simulink model "testVPSdriver"  (R2015b)
settings: Solver=VariableStepAuto  StartTime=0.0  StopTime=inf  RelTol=1e-3
libraries: robotlib x2
settings Model: Creator=exbot  LastModifiedBy=exbot

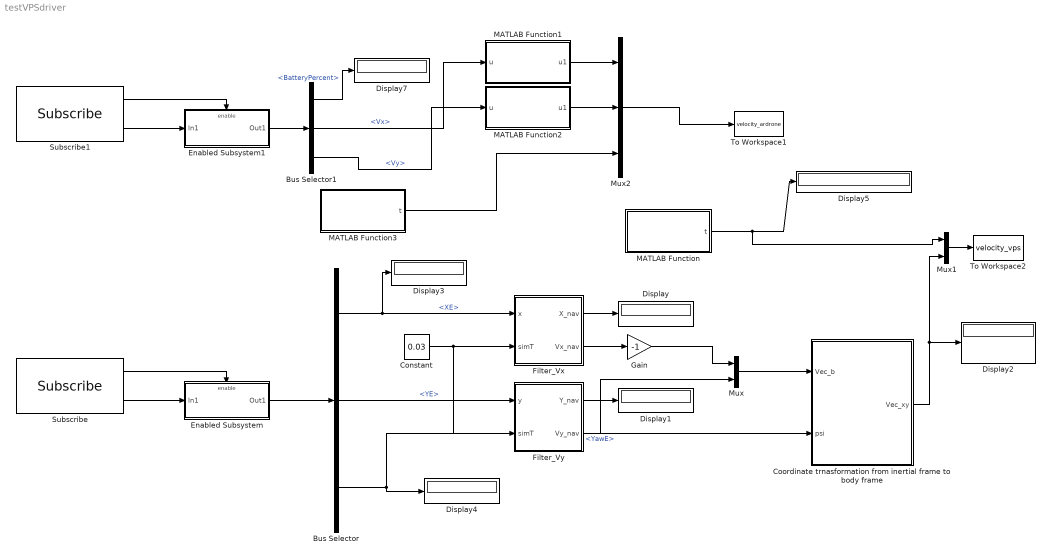
== system testVPSdriver ==
  Bus Selector : BusSelector  OutputSignals=XE,YE,YawE
  Bus Selector1 : BusSelector  OutputSignals=BatteryPercent,Vx,Vy
  Constant : Constant  Value=0.03
  "Coordinate trnasformation from inertial frame to body frame " : MATLAB Function  TreatAsAtomicUnit=on
  Display{,1..5,7} (7 alike) : Display
  Enabled Subsystem : Subsystem  TreatAsAtomicUnit=on
  Enabled Subsystem1 : Subsystem  TreatAsAtomicUnit=on
  Filter_Vx : MATLAB Function  TreatAsAtomicUnit=on
  Filter_Vy : MATLAB Function  TreatAsAtomicUnit=on
  Gain : Gain  Gain=-1
  MATLAB Function : MATLAB Function  TreatAsAtomicUnit=on
  MATLAB Function1 : MATLAB Function  TreatAsAtomicUnit=on
  MATLAB Function2 : MATLAB Function  TreatAsAtomicUnit=on
  MATLAB Function3 : MATLAB Function  TreatAsAtomicUnit=on
  Mux : Mux  Inputs=2
  Mux1 : Mux  Inputs=2
  Mux2 : Mux  Inputs=3
  Subscribe : robotlib/Subscribe  SourceLibraryInfo=This block requires Robotics System Toolbox  topicSource=Select from ROS network  topic=/vpsnavdata  messageType=vps_driver/vps_navdata  sampleTime=-1  messageQueueLength=1
  Subscribe1 : robotlib/Subscribe  SourceLibraryInfo=This block requires Robotics System Toolbox  topicSource=Select from ROS network  topic=/ardrone/navdata  messageType=ardrone_autonomy/Navdata  sampleTime=-1  messageQueueLength=1
  To Workspace1 : ToWorkspace  VariableName=velocity_ardrone  SampleTime=-1
  To Workspace2 : ToWorkspace  VariableName=velocity_vps  SampleTime=-1
  wires:
  Subscribe/2 -> Enabled Subsystem/1(In1)
  Subscribe/1 -> Enabled Subsystem/Enable
  Bus Selector/1 -> Display3/1, Filter_Vx/1(x)  "<XE>"
  Bus Selector/2 -> Filter_Vy/1(y)  "<YE>"
  Enabled Subsystem/1(Out1) -> Bus Selector/1
  Subscribe1/2 -> Enabled Subsystem1/1(In1)
  Subscribe1/1 -> Enabled Subsystem1/Enable
  Enabled Subsystem1/1(Out1) -> Bus Selector1/1
  Bus Selector1/1 -> Display7/1  "<BatteryPercent>"
  Bus Selector1/2 -> MATLAB Function1/1(u)  "<Vx>"
  Bus Selector1/3 -> MATLAB Function2/1(u)  "<Vy>"
  Mux2/1 -> To Workspace1/1
  Bus Selector/3 -> "Coordinate trnasformation from inertial frame to body frame "/2(psi), Display4/1  "<YawE>"
  Filter_Vx/1(X_nav) -> Display/1
  Filter_Vy/1(Y_nav) -> Display1/1
  Mux/1 -> "Coordinate trnasformation from inertial frame to body frame "/1(Vec_b)
  Filter_Vx/2(Vx_nav) -> Gain/1
  Filter_Vy/2(Vy_nav) -> Mux/2
  Constant/1 -> Filter_Vy/2(simT), Filter_Vx/2(simT)
  MATLAB Function/1(t) -> Mux1/1, Display5/1
  "Coordinate trnasformation from inertial frame to body frame "/1(Vec_xy) -> Mux1/2, Display2/1
  Mux1/1 -> To Workspace2/1
  MATLAB Function3/1(t) -> Mux2/3
  MATLAB Function1/1(u1) -> Mux2/1
  MATLAB Function2/1(u1) -> Mux2/2
  Gain/1 -> Mux/1

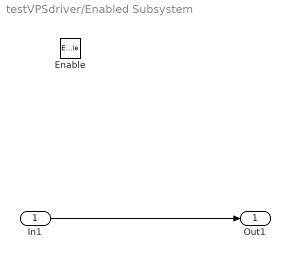
== system testVPSdriver/Enabled Subsystem ==
  In1 : Inport
  Enable : EnablePort
  Out1 : Outport
  wires:
  In1/1 -> Out1/1

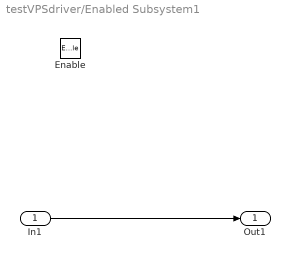
== system testVPSdriver/Enabled Subsystem1 ==
  In1 : Inport
  Enable : EnablePort
  Out1 : Outport
  wires:
  In1/1 -> Out1/1

== matlab function testVPSdriver/Coordinate trnasformation from inertial frame to body frame  ==
  data: Vec_b input; Vec_xy output; psi input
function Vec_xy  = fcn(Vec_b , psi)
%#codegen
T = [cos(psi) sin(psi) ; sin(psi) -cos(psi)] ; 
Vec_xy = T*Vec_b(1:2,1);

== matlab function testVPSdriver/MATLAB Function ==
  data: t output
function t = sysTime( )
coder.extrinsic('now');
t = 0;
t = now;
end

== matlab function testVPSdriver/Filter_Vx ==
  data: x input; X_nav output; Vx_nav output; simT input
function [X_nav,Vx_nav] = fcn(x,simT)
persistent Phi;
if isempty(Phi)
    Phi = [1 simT;0 1];
end

persistent Tao;
if isempty(Tao)
    Tao = [0 simT]';
end

persistent Q;
if isempty(Q)
    Q = 50;
end

persistent H;
if isempty(H)
    H = [1 0];
end

persistent R;
if isempty(R)
    R = 7.81e-1;
end

persistent Xe;
if isempty(Xe)
    Xe = [0 0]';
end

persistent X_e;
if isempty(X_e)
    X_e = [0 0]';
end

persistent Z_e;
if isempty(Z_e)
    Z_e = 0;
end

persistent P;
if isempty(P)
    P = Q*[1 0;0 1]; % 估计误差协方差阵
end

persistent P_;
if isempty(P_)
    P_ = Q*[1 0;0 1]; % 估计误差协方差阵
end

% 状态变量的先验估计
X_e = Phi*Xe;
% 观测向量的先验估计
Z_e = H*X_e;
% 计算先验估计误差协方差阵
P_ = Phi*P*Phi'+Tao*Q*Tao';

% 观测值 [x y z yaw]'  输入Z=[x y z pitch yaw roll vx vy vz]'
Zm = x/1000.0;

% 计算卡尔曼增益
Kk = P_*H'*(inv(H*P_*H'+R));
% 计算后验估计
Xe = X_e+Kk*(Zm-Z_e);
% 计算后验协方差阵
P=(eye(2)-Kk*H)*P_;

X_nav = Xe(1);
Vx_nav = Xe(2);
end

== matlab function testVPSdriver/Filter_Vy ==
  data: y input; Y_nav output; Vy_nav output; simT input
function [Y_nav,Vy_nav] = fcn(y,simT)
persistent Phi;
if isempty(Phi)
    Phi = [1 simT;0 1];
end

persistent Tao;
if isempty(Tao)
    Tao = [0 simT]';
end

persistent Q;
if isempty(Q)
    Q = 50;
end

persistent H;
if isempty(H)
    H = [1 0];
end

persistent R;
if isempty(R)
    R = 2.33e-1;
end

persistent Xe;
if isempty(Xe)
    Xe = [0 0]';
end

persistent X_e;
if isempty(X_e)
    X_e = [0 0]';
end

persistent Z_e;
if isempty(Z_e)
    Z_e = 0;
end

persistent P;
if isempty(P)
    P = Q*[1 0;0 1]; % 估计误差协方差阵
end

persistent P_;
if isempty(P_)
    P_ = Q*[1 0;0 1]; % 估计误差协方差阵
end

% 状态变量的先验估计
X_e = Phi*Xe;
% 观测向量的先验估计
Z_e = H*X_e;
% 计算先验估计误差协方差阵
P_ = Phi*P*Phi'+Tao*Q*Tao';

% 观测值 [x y z yaw]'  输入Z=[x y z pitch yaw roll vx vy vz]'
Zm = y/1000.0;

% 计算卡尔曼增益
Kk = P_*H'*(inv(H*P_*H'+R));
% 计算后验估计
Xe = X_e+Kk*(Zm-Z_e);
% 计算后验协方差阵
P=(eye(2)-Kk*H)*P_;

Y_nav = Xe(1);
Vy_nav = Xe(2);
end

== matlab function testVPSdriver/MATLAB Function2 ==
  data: u1 output; u input
function u1 = s2d( u )
u1 = 0;
u1 = double(u);
end

== matlab function testVPSdriver/MATLAB Function3 ==
  data: t output
function t = sysTime( )
coder.extrinsic('now');
t = 0;
t = now;
end

== matlab function testVPSdriver/MATLAB Function1 ==
  data: u1 output; u input
function u1 = s2d( u )
u1 = 0;
u1 = double(u);
end
